simulink model "NeuromuscularModel_3R60_2D"  (R2019b)
settings: Solver=ode15s  StartTime=0.0  StopTime=30  MaxStep=.01  RelTol=1e-4  AbsTol=1e-6  EnableMultiTasking=on
values from neighbouring files (symbols this model uses):
  dt_visual = 1/50    (= 0.02)    [evaluateCost.m]    (also in optimize.m = 0.0333333333333)
  initialTargetAngle = 70*pi/180    (= 1.2217304764)    [setInit.m]
  LongDelay = 0.020    (= 0.02)    [ControlParams.m]
  LPreStimBFSHst = Gains(51)    [assignGains.m]
  LPreStimGASst = Gains(52)    [assignGains.m]
  LPreStimGLUst = Gains(47)    [assignGains.m]
  LPreStimHAMst = Gains(48)    [assignGains.m]
  LPreStimHFLst = Gains(46)    [assignGains.m]
  LPreStimRFst = Gains(49)    [assignGains.m]
  LPreStimSOLst = Gains(53)    [assignGains.m]
  LPreStimTAst = Gains(54)    [assignGains.m]
  LPreStimVASst = Gains(50)    [assignGains.m]
  MidDelay = 0.010    (= 0.01)    [ControlParams.m]
  RPreStimGLUsw = Gains(95)    [assignGains.m]
  RPreStimHAMsw = Gains(96)    [assignGains.m]
  RPreStimHFLsw = Gains(94)    [assignGains.m]
  RPreStimRFsw = Gains(97)    [assignGains.m]
  ShortDelay = 0.005    [ControlParams.m]
  termination_height = 0.5    [ControlParams.m]
  vy0 = paramIC(10)*.2    [setInit.m]
undefined symbols (not defined in the file or in its folder): g, hatLeftHipToCenterDistWidth, hatLeftHipToCG, initialTargetAngleR, LongLoopDelay, LPreStimHABst, LPreStimHADst, magnitude, obstacle_depth, obstacle_height, obstacle_width, obstacle_x, RPreStimHABsw, RPreStimHADsw, thetaHATref, X, Y, y0, Z
libraries: NeuroMuscularLibrary x100, sm_lib x24, nesl_utility x16, simulink x5
(part 3 of 4)

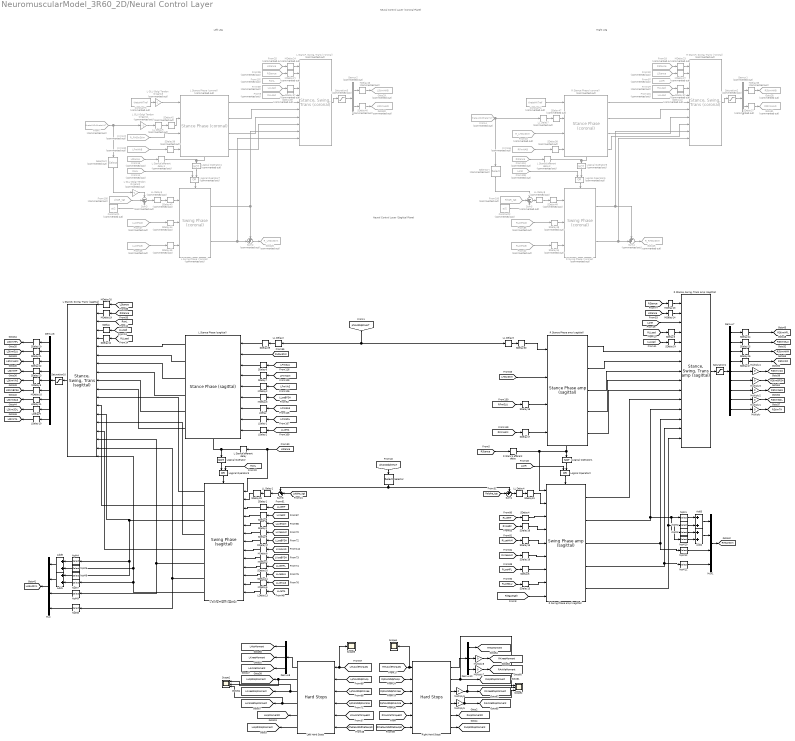
== system NeuromuscularModel_3R60_2D/Neural Control Layer ==
  note: Neural Control Layer
      | (Sagittal Plane)
  note: Neural Control Layer
      | (Coronal Plane)
  note: Right Leg
  note: Left Leg
  Add{1..3,9} (4 alike) : Sum  Inputs=2
  Constant1 : Constant  Commented=on  Value=pi/2
  Constant2 : Constant  Commented=on  Value=pi/2
  Constant3 : Constant  Commented=on  Value=thetaHATref
  Constant4 : Constant  Commented=on  Value=thetaHATref
  Demux1 : Demux  Commented=on  Outputs=2
  Demux10 : Demux  Outputs=3
  Demux2 : Demux  Commented=on  Outputs=2
  Demux6 : Demux  Outputs=9
  Demux7 : Demux  Outputs=9
  Demux8 : Demux  Outputs=3
  From100 : From  Commented=on  GotoTag=RhipR_tgt  TagVisibility=global
      settings: CloseFcn=tagdialog Close
  From101 : From  Commented=on  GotoTag=LLLoad  TagVisibility=global
      settings: CloseFcn=tagdialog Close
  From102 : From  Commented=on  GotoTag=RonL  TagVisibility=global
      settings: CloseFcn=tagdialog Close
  From105 : From  Commented=on  GotoTag=LhipR_tgt  TagVisibility=global
      settings: CloseFcn=tagdialog Close
  From108 : From  Commented=on  GotoTag=LonR  TagVisibility=global
      settings: CloseFcn=tagdialog Close
  From11 : From  Commented=on  GotoTag=RonL  TagVisibility=global
      settings: CloseFcn=tagdialog Close
  From110 : From  Commented=on  GotoTag=RStance  TagVisibility=global
      settings: CloseFcn=tagdialog Close
  From15 : From  Commented=on  GotoTag=LStance  TagVisibility=global
      settings: CloseFcn=tagdialog Close
  From16 : From  Commented=on  GotoTag=R_LHSwStim  TagVisibility=global
      settings: CloseFcn=tagdialog Close
  From18 : From  Commented=on  GotoTag=RStance  TagVisibility=global
      settings: CloseFcn=tagdialog Close
  From22 : From  Commented=on  GotoTag=RLceHAB  TagVisibility=global
      settings: CloseFcn=tagdialog Close
  From23 : From  Commented=on  GotoTag=R_RHSwStim  TagVisibility=global
      settings: CloseFcn=tagdialog Close
  From25 : From  Commented=on  GotoTag=LStance  TagVisibility=global
      settings: CloseFcn=tagdialog Close
  From26 : From  Commented=on  GotoTag=LLceHAB  TagVisibility=global
      settings: CloseFcn=tagdialog Close
  From27 : From  Commented=on  GotoTag=LLceHAD  TagVisibility=global
      settings: CloseFcn=tagdialog Close
  From29 : From  Commented=on  GotoTag=RLLoad  TagVisibility=global
      settings: CloseFcn=tagdialog Close
  From32 : From  Commented=on  GotoTag=LStance  TagVisibility=global
      settings: CloseFcn=tagdialog Close
  From4 : From  Commented=on  GotoTag=thetaANDdthetaHAT  TagVisibility=global
  From7 : From  Commented=on  GotoTag=thetaANDdthetaHAT  TagVisibility=global
  From85 : From  Commented=on  GotoTag=RLceHAD  TagVisibility=global
      settings: CloseFcn=tagdialog Close
  From88 : From  Commented=on  GotoTag=LLLoad  TagVisibility=global
      settings: CloseFcn=tagdialog Close
  From9 : From  Commented=on  GotoTag=RLLoad  TagVisibility=global
      settings: CloseFcn=tagdialog Close
  From94 : From  Commented=on  GotoTag=RFmHAB  TagVisibility=global
      settings: CloseFcn=tagdialog Close
  From95 : From  Commented=on  GotoTag=RStance  TagVisibility=global
      settings: CloseFcn=tagdialog Close
  From97 : From  Commented=on  GotoTag=LonR  TagVisibility=global
      settings: CloseFcn=tagdialog Close
  From99 : From  Commented=on  GotoTag=LFmHAB  TagVisibility=global
      settings: CloseFcn=tagdialog Close
  Goto25 : Goto  Commented=on  GotoTag=R_RHSwStim  TagVisibility=global
  Goto26 : Goto  Commented=on  GotoTag=R_LHSwStim  TagVisibility=global
  Goto28 : Goto  Commented=on  GotoTag=RStimHAB  TagVisibility=global
  Goto29 : Goto  Commented=on  GotoTag=LStimHAB  TagVisibility=global
  Goto30 : Goto  Commented=on  GotoTag=LStimHAD  TagVisibility=global
  Goto31 : Goto  Commented=on  GotoTag=RStimHAD  TagVisibility=global
  L GLU Golgi Tendon Organs1 : Gain  Commented=on  Gain=-1
  L GLU Golgi Tendon Organs2 : Gain  Commented=on  Gain=-1
  L GLU Golgi Tendon Organs3 : Gain  Commented=on  Gain=-1
  L Stance afferent delay : TransportDelay  DelayTime=MidDelay
  L Stance afferent delay1 : TransportDelay  Commented=on  DelayTime=MidDelay
  L Stance afferent delay2 : TransportDelay  Commented=on  DelayTime=MidDelay
  L Stance Phase (coronal) : NeuroMuscularLibrary/Stance Phase (coronal)  Commented=on  PreStimHABst=LPreStimHABst  PreStimHADst=LPreStimHADst  GainFHABst=LGainFHABst  GainPhiHATHABst=LGainPhiHATHABst  GainDphiHATHABst=LGainDphiHATHABst  GainPhiHATHADst=LGainPhiHATHADst  GainDphiHATHADst=LGainDphiHATHADst  GainSHABcHABst=LGainSHABcHABst  GainSHADcHADst=LGainSHADcHADst
  L Stance Phase (sagittal) : NeuroMuscularLibrary/Stance Phase (sagittal)  PreStimHFLst=LPreStimHFLst  PreStimGLUst=LPreStimGLUst  PreStimHAMst=LPreStimHAMst  PreStimRFst=LPreStimRFst  PreStimVASst=LPreStimVASst  PreStimBFSHst=LPreStimBFSHst  PreStimGASst=LPreStimGASst  PreStimSOLst=LPreStimSOLst  PreStimTAst=LPreStimTAst  GainFGLUst=LGainFGLUst  GainFVASst=LGainFVASst  GainFSOLst=LGainFSOLst  GainFHAMst=LGainFHAMst  LceOffsetBFSHVASst=LLceOffsetBFSHVASst  GainLBFSHVASst=LGainLBFSHVASst  LceOffsetBFSHst=LLceOffsetBFSHst  GainLBFSHst=LGainLBFSHst  GainFGASst=LGainFGASst  phiHATref=phiHATref  GainPhiHATHFLst=LGainPhiHATHFLst  GainDphiHATHFLst=LGainDphiHATHFLst  GainPhiHATGLUst=LGainPhiHATGLUst  GainDphiHATGLUst=LGainDphiHATGLUst  GainSGLUHAMst=LGainSGLUHAMst  GainSGLUcHFLst=LGainSGLUcHFLst  GainSHAMcHFLst=LGainSHAMcHFLst  GainSHFLcGLUst=LGainSHFLcGLUst  GainSRFcGLUst=LGainSRFcGLUst  LceOffsetTAst=LLceOffsetTAst  GainLTAst=LGainLTAst  GainFSOLTAst=LGainFSOLTAst
  "L Stance, Swing, Trans (coronal)" : NeuroMuscularLibrary/Stance, Swing, Trans (coronal)  Commented=on  transSupst_C=LtransSupst_C  transsw_C=Ltranssw_C
  "L Stance, Swing, Trans (sagittal)" : NeuroMuscularLibrary/Stance, Swing, Trans (sagittal)  transSupst=LtransSupst  transsw=Ltranssw
  L Swing Phase (coronal) : NeuroMuscularLibrary/Swing Phase (coronal)  Commented=on  PreStimHABsw=LPreStimHABsw  PreStimHADsw=LPreStimHADsw  GainLHABsw=LGainLHABsw  GainLHADsw=LGainLHADsw
  L Swing Phase (sagittal) : NeuroMuscularLibrary/Swing Phase (sagittal)  PreStimHFLsw=LPreStimHFLsw  PreStimGLUsw=LPreStimGLUsw  PreStimHAMsw=LPreStimHAMsw  PreStimRFsw=LPreStimRFsw  PreStimVASsw=LPreStimVASsw  PreStimBFSHsw=LPreStimBFSHsw  PreStimGASsw=LPreStimGASsw  PreStimSOLsw=LPreStimSOLsw  PreStimTAsw=LPreStimTAsw  GainLTAsw=LGainLTAsw  LceOffsetTAsw=LLceOffsetTAsw  GainLRFHFLsw=LGainLRFHFLsw  GainVRFHFLsw=LGainVRFHFLsw  GainLHAMGLUsw=LGainLHAMGLUsw  GainVHAMGLUsw=LGainVHAMGLUsw  GainVRFBFSHsw=LGainVRFBFSHsw  GainVVASRFsw=LGainVVASRFsw  GainVBFSHsw=LGainVBFSHsw  GainLHAMsw=LGainLHAMsw  GainSHAMBFSHsw=LGainSHAMBFSHsw  GainSHAMGASsw=LGainSHAMGASsw  SHAMthresholdsw=LSHAMthresholdsw  GainLHFLsw=LGainLHFLsw  GainLGLUsw=LGainLGLUsw  LceOffsetVASsw=LLceOffsetVASsw  GainLVASsw=LGainLVASsw  legLengthClr=LlegLengthClr  deltaLegAngleThr=LdeltaLegAngleThr
  LDelay : TransportDelay  DelayTime=LongDelay
  LDelay1 : TransportDelay  DelayTime=LongDelay
  LDelay10 : TransportDelay  DelayTime=LongDelay  InitialOutput=LPreStimTAst
  LDelay11 : TransportDelay  DelayTime=LongDelay  InitialOutput=LPreStimGASst
  LDelay13 : TransportDelay  DelayTime=LongDelay  InitialOutput=1
  LDelay2 : TransportDelay  DelayTime=LongDelay  InitialOutput=1
  LDelay9 : TransportDelay  DelayTime=LongDelay  InitialOutput=LPreStimSOLst
  LL Delay1 : TransportDelay  DelayTime=LongLoopDelay/2  InitialOutput=initialTargetAngle
  LL Delay2 : TransportDelay  DelayTime=LongLoopDelay/2
  LL Delay3 : TransportDelay  DelayTime=LongLoopDelay/2
  LL Delay4 : TransportDelay  DelayTime=LongLoopDelay/2  InitialOutput=initialTargetAngle
  LL Delay5 : TransportDelay  Commented=on  DelayTime=LongLoopDelay/2  InitialOutput=initialTargetAngleR
  LL Delay6 : TransportDelay  Commented=on  DelayTime=LongLoopDelay/2
  LL Delay7 : TransportDelay  Commented=on  DelayTime=LongLoopDelay/2
  LL Delay8 : TransportDelay  Commented=on  DelayTime=LongLoopDelay/2  InitialOutput=initialTargetAngleR
  Left Hard Stops : NeuroMuscularLibrary/Hard Stops  SystemSampleTime=-1  Latency=0  AutoFrameSizeCalculation=off
  Logical Operator : Logic  Operator=NOT  AllPortsSameDT=off  OutDataTypeStr=boolean
  Logical Operator1 : Logic  Operator=NOT  AllPortsSameDT=off  OutDataTypeStr=boolean
  Logical Operator2 : Logic  Operator=OR  AllPortsSameDT=off  OutDataTypeStr=boolean
  Logical Operator3 : Logic  Operator=OR  AllPortsSameDT=off  OutDataTypeStr=boolean
  Logical Operator4 : Logic  Commented=on  Operator=NOT  AllPortsSameDT=off  OutDataTypeStr=boolean
  Logical Operator5 : Logic  Commented=on  Operator=NOT  AllPortsSameDT=off  OutDataTypeStr=boolean
  Logical Operator6 : Logic  Commented=on  Operator=OR  AllPortsSameDT=off  OutDataTypeStr=boolean
  Logical Operator7 : Logic  Commented=on  Operator=OR  AllPortsSameDT=off  OutDataTypeStr=boolean
  MDelay10 : TransportDelay  DelayTime=MidDelay  InitialOutput=LPreStimBFSHst
  MDelay{2,4,8,13..14,19..20} (7 alike) : TransportDelay  DelayTime=MidDelay
  MDelay17 : TransportDelay  DelayTime=MidDelay  InitialOutput=1
  MDelay{21..24} (4 alike) : TransportDelay  Commented=on  DelayTime=MidDelay
  MDelay3 : TransportDelay  DelayTime=MidDelay  InitialOutput=1
  MDelay5 : TransportDelay  DelayTime=MidDelay  InitialOutput=1
  MDelay9 : TransportDelay  DelayTime=MidDelay  InitialOutput=LPreStimVASst
  Multiply{,1..8} (9 alike) : Gain  Gain=0
  Mux : Mux
  Mux1 : Mux
  R Stance afferent delay : TransportDelay  DelayTime=MidDelay
  R Stance Phase (coronal) : NeuroMuscularLibrary/Stance Phase (coronal)  Commented=on  PreStimHABst=RPreStimHABst  PreStimHADst=RPreStimHADst  GainFHABst=RGainFHABst  GainPhiHATHABst=RGainPhiHATHABst  GainDphiHATHABst=RGainDphiHATHABst  GainPhiHATHADst=RGainPhiHATHADst  GainDphiHATHADst=RGainDphiHATHADst  GainSHABcHABst=RGainSHABcHABst  GainSHADcHADst=RGainSHADcHADst
  R Stance Phase amp (sagittal) : NeuroMuscularLibrary/Stance Phase amp (sagittal)  PreStimHFLst=RPreStimHFLst  PreStimGLUst=RPreStimGLUst  PreStimHAMst=RPreStimHAMst  PreStimRFst=RPreStimRFst  GainFGLUst=RGainFGLUst  GainFHAMst=RGainFHAMst  phiHATref=phiHATref  GainPhiHATHFLst=RGainPhiHATHFLst  GainDphiHATHFLst=RGainDphiHATHFLst  GainPhiHATGLUst=RGainPhiHATGLUst  GainDphiHATGLUst=RGainDphiHATGLUst  GainSGLUHAMst=RGainSGLUHAMst  GainSGLUcHFLst=RGainSGLUcHFLst  GainSHAMcHFLst=RGainSHAMcHFLst  GainSHFLcGLUst=RGainSHFLcGLUst  GainSRFcGLUst=RGainSRFcGLUst
  "R Stance, Swing, Trans (coronal)" : NeuroMuscularLibrary/Stance, Swing, Trans (coronal)  Commented=on  transSupst_C=RtransSupst_C  transsw_C=Rtranssw_C
  "R Stance, Swing, Trans amp (sagittal)" : NeuroMuscularLibrary/Stance, Swing, Trans amp (sagittal)  transSupst=RtransSupst  transsw=Rtranssw
  R Swing Phase (coronal) : NeuroMuscularLibrary/Swing Phase (coronal)  Commented=on  PreStimHABsw=RPreStimHABsw  PreStimHADsw=RPreStimHADsw  GainLHABsw=RGainLHABsw  GainLHADsw=RGainLHADsw
  R Swing Phase amp (sagittal) : NeuroMuscularLibrary/Swing Phase amp (sagittal)  PreStimHFLsw=RPreStimHFLsw  PreStimGLUsw=RPreStimGLUsw  PreStimHAMsw=RPreStimHAMsw  PreStimRFsw=RPreStimRFsw  GainLRFHFLsw=RGainLRFHFLsw  GainVRFHFLsw=RGainVRFHFLsw  GainLHAMGLUsw=RGainLHAMGLUsw  GainVHAMGLUsw=RGainVHAMGLUsw  GainLHAMsw=RGainLHAMsw  GainLHFLsw=RGainLHFLsw  GainLGLUsw=RGainLGLUsw  legLengthClr=RlegLengthClr  deltaLegAngleThr=RdeltaLegAngleThr
  Right Hard Stops : NeuroMuscularLibrary/Hard Stops  SystemSampleTime=-1  Latency=0  AutoFrameSizeCalculation=off
  SDelay{,3,6..9,12,14,16..19,29..30} (14 alike) : TransportDelay  DelayTime=ShortDelay
  SDelay{1..2,4..5,10..11,13,15} (8 alike) : TransportDelay  DelayTime=ShortDelay  InitialOutput=1
  SDelay20 : TransportDelay  DelayTime=ShortDelay  InitialOutput=LPreStimHFLst
  SDelay21 : TransportDelay  DelayTime=ShortDelay  InitialOutput=LPreStimGLUst
  SDelay22 : TransportDelay  DelayTime=ShortDelay  InitialOutput=LPreStimHAMst
  SDelay23 : TransportDelay  DelayTime=ShortDelay  InitialOutput=LPreStimRFst
  SDelay24 : TransportDelay  DelayTime=ShortDelay  InitialOutput=RPreStimHFLsw
  SDelay25 : TransportDelay  DelayTime=ShortDelay  InitialOutput=RPreStimGLUsw
  SDelay26 : TransportDelay  DelayTime=ShortDelay  InitialOutput=RPreStimHAMsw
  SDelay27 : TransportDelay  DelayTime=ShortDelay  InitialOutput=RPreStimRFsw
  SDelay28 : TransportDelay  DelayTime=ShortDelay  InitialOutput=initialTargetAngle
  SDelay31 : TransportDelay  DelayTime=ShortDelay  InitialOutput=initialTargetAngle
  SDelay{32..33,36,38..39,41..42,47} (8 alike) : TransportDelay  Commented=on  DelayTime=ShortDelay
  SDelay{34,44..45,49} (4 alike) : TransportDelay  Commented=on  DelayTime=ShortDelay  InitialOutput=1
  SDelay35 : TransportDelay  Commented=on  DelayTime=ShortDelay  InitialOutput=RPreStimHABsw
  SDelay37 : TransportDelay  Commented=on  DelayTime=ShortDelay  InitialOutput=RPreStimHADsw
  SDelay40 : TransportDelay  Commented=on  DelayTime=ShortDelay  InitialOutput=LPreStimHADst
  SDelay43 : TransportDelay  Commented=on  DelayTime=ShortDelay  InitialOutput=initialTargetAngleR
  SDelay46 : TransportDelay  Commented=on  DelayTime=ShortDelay  InitialOutput=LPreStimHABst
  SDelay48 : TransportDelay  Commented=on  DelayTime=ShortDelay  InitialOutput=initialTargetAngleR
  Saturation1 : Saturate  UpperLimit=1  LowerLimit=0.01  ZeroCross=off
  Saturation10 : Saturate  UpperLimit=1  LowerLimit=0.01  ZeroCross=off
  Saturation2 : Saturate  Commented=on  UpperLimit=1  LowerLimit=0.01  ZeroCross=off
  Saturation3 : Saturate  Commented=on  UpperLimit=1  LowerLimit=0.01  ZeroCross=off
  Scope1 : Scope  NumInputPorts=3
  Scope2 : Scope  NumInputPorts=3
  Scope3 : Scope
  Scope4 : Scope
  Selector : Selector  InputPortWidth=2  IndexOptions=Index vector (dialog)  Indices=[1]  OutputSizes=1
  Selector1 : Selector  Commented=on  InputPortWidth=2  IndexOptions=Index vector (dialog)  Indices=[1]  OutputSizes=1
  Selector2 : Selector  Commented=on  InputPortWidth=2  IndexOptions=Index vector (dialog)  Indices=[1]  OutputSizes=1
  Sum1 : Sum  Inputs=-+|
  Sum2 : Sum  Commented=on  Inputs=++|
  Sum3 : Sum  Commented=on  Inputs=--+
  Sum4 : Sum  Commented=on  Inputs=++|
  Sum5 : Sum  Commented=on  Inputs=--+
  Sum6 : Sum  Inputs=-+|
  hipM{1,4,9,12} (4 alike) : Selector  InputPortWidth=2  IndexOptions=Index vector (dialog)  Indices=1  OutputSizes=1
  hipM10 : Selector  InputPortWidth=3  IndexOptions=Index vector (dialog)  Indices=2  OutputSizes=1
  hipM{2,5,8,11} (4 alike) : Selector  InputPortWidth=3  IndexOptions=Index vector (dialog)  Indices=1  OutputSizes=1
  hipM3 : Selector  InputPortWidth=2  IndexOptions=Index vector (dialog)  Indices=2  OutputSizes=1
  hipM6 : Selector  InputPortWidth=2  IndexOptions=Index vector (dialog)  Indices=2  OutputSizes=1
  hipM7 : Selector  InputPortWidth=3  IndexOptions=Index vector (dialog)  Indices=2  OutputSizes=1
  tag scope: LAnkleMoment=global, LAnkleStopMoment=global, LHSwStim=global, LHipMoment=global, LHipMomentR=global, LHipRStopMoment=global, LHipStopMoment=global, LKneeMoment=global, LKneeStopMoment=global, LStimBFSH=global, LStimGAS=global, LStimGLU=global, LStimHAM=global, LStimHFL=global, LStimRF=global, LStimSOL=global, LStimTA=global, LStimVAS=global, RAnkleMoment=global, RAnkleStopMoment=global, RHSwStim=global, RHipMoment=global, RHipMomentR=global, RHipRStopMoment=global, RHipStopMoment=global, RKneeMoment=global, RKneeStopMoment=global, RStimBFSH=global, RStimGAS=global, RStimGLU=global, RStimHAM=global, RStimHFL=global, RStimRF=global, RStimSOL=global, RStimTA=global, RStimVAS=global
  wires:
  LDelay11/1 -> [LStimGAS]
  LDelay10/1 -> [LStimTA]
  L Swing Phase (sagittal)/7 -> "L Stance, Swing, Trans (sagittal)"/18, hipM8/1
  Mux/1 -> [LHSwStim]
  hipM2/1 -> Add3/2
  SDelay11/1 -> L Swing Phase (sagittal)/11
  SDelay24/1 -> [RStimHFL]
  [RLceRF] -> SDelay4/1
  MDelay19/1 -> "L Stance, Swing, Trans (sagittal)"/2
  SDelay10/1 -> L Swing Phase (sagittal)/10
  hipM10/1 -> Add2/2
  R Stance Phase amp (sagittal)/5 -> "R Stance, Swing, Trans amp (sagittal)"/10
  hipM4/1 -> Add9/1
  SDelay2/1 -> L Swing Phase (sagittal)/5
  [RLceGLU] -> SDelay13/1
  L Swing Phase (sagittal)/1 -> "L Stance, Swing, Trans (sagittal)"/12
  LDelay/1 -> L Stance Phase (sagittal)/7
  L Stance Phase (sagittal)/1 -> "L Stance, Swing, Trans (sagittal)"/6
  SDelay9/1 -> L Swing Phase (sagittal)/6
  L Swing Phase (sagittal)/3 -> "L Stance, Swing, Trans (sagittal)"/14, hipM6/1, hipM4/1
  R Swing Phase amp (sagittal)/4 -> "R Stance, Swing, Trans amp (sagittal)"/14, hipM11/1
  Add2/1 -> Mux1/2
  L Swing Phase (sagittal)/5 -> "L Stance, Swing, Trans (sagittal)"/16
  SDelay14/1 -> "R Stance, Swing, Trans amp (sagittal)"/5
  Demux6/2 -> SDelay21/1
  R Stance Phase amp (sagittal)/2 -> "R Stance, Swing, Trans amp (sagittal)"/7
  SDelay12/1 -> "L Stance, Swing, Trans (sagittal)"/5
  MDelay2/1 -> L Stance Phase (sagittal)/5
  Sum1/1 -> LL Delay4/1
  hipM6/1 -> Add1/1
  R Stance Phase amp (sagittal)/3 -> "R Stance, Swing, Trans amp (sagittal)"/8
  LDelay9/1 -> [LStimSOL]
  Demux6/1 -> SDelay20/1
  L Stance Phase (sagittal)/6 -> "L Stance, Swing, Trans (sagittal)"/11
  SDelay4/1 -> R Swing Phase amp (sagittal)/3
  hipM11/1 -> Mux1/4
  MDelay8/1 -> L Swing Phase (sagittal)/8
  Add3/1 -> Mux1/1
  R Swing Phase amp (sagittal)/3 -> "R Stance, Swing, Trans amp (sagittal)"/13, hipM12/1
  "R Stance, Swing, Trans amp (sagittal)"/1 -> Saturation1/1
  Add1/1 -> Mux/2
  hipM9/1 -> Mux/3
  L Stance Phase (sagittal)/3 -> "L Stance, Swing, Trans (sagittal)"/8
  Demux7/8 -> Multiply1/1
  Logical Operator2/1 -> R Swing Phase amp (sagittal)/Enable
  hipM5/1 -> Add9/2
  MDelay20/1 -> "L Stance, Swing, Trans (sagittal)"/1
  L Swing Phase (sagittal)/2 -> "L Stance, Swing, Trans (sagittal)"/13
  hipM8/1 -> Mux/4
  L Swing Phase (sagittal)/4 -> "L Stance, Swing, Trans (sagittal)"/15
  L Swing Phase (sagittal)/8 -> "L Stance, Swing, Trans (sagittal)"/19, hipM5/1, hipM7/1
  [LStance] -> MDelay20/1
  R Stance Phase amp (sagittal)/4 -> "R Stance, Swing, Trans amp (sagittal)"/9
  LL Delay3/1 -> SDelay30/1
  SDelay30/1 -> R Stance Phase amp (sagittal)/1
  SDelay22/1 -> [LStimHAM]
  SDelay29/1 -> L Stance Phase (sagittal)/1
  SDelay28/1 -> L Swing Phase (sagittal)/2
  hipM1/1 -> Add3/1
  R Swing Phase amp (sagittal)/5 -> "R Stance, Swing, Trans amp (sagittal)"/15, hipM2/1, hipM10/1
  Sum6/1 -> LL Delay1/1
  Demux7/1 -> SDelay24/1
  [LLceGLU] -> SDelay11/1
  [RLceHFL] -> SDelay5/1
  LL Delay4/1 -> SDelay31/1
  L Stance Phase (sagittal)/2 -> "L Stance, Swing, Trans (sagittal)"/7
  R Stance Phase amp (sagittal)/1 -> "R Stance, Swing, Trans amp (sagittal)"/6
  [LLceVAS] -> MDelay5/1
  [LHSwStim] -> R Stance Phase amp (sagittal)/2
  SDelay/1 -> "L Stance, Swing, Trans (sagittal)"/4
  SDelay27/1 -> [RStimRF]
  Demux7/6 -> Multiply3/1
  MDelay10/1 -> [LStimBFSH]
  Add9/1 -> Mux/1
  [LLceHFL] -> SDelay10/1
  SDelay26/1 -> [RStimHAM]
  SDelay21/1 -> [LStimGLU]
  [LLLoad] -> SDelay14/1
  Saturation1/1 -> Demux7/1
  SDelay5/1 -> R Swing Phase amp (sagittal)/7
  [LFmSOL] -> LDelay1/1
  hipM12/1 -> Mux1/3
  [LonR] -> "R Stance, Swing, Trans amp (sagittal)"/3
  [LLLoad] -> SDelay/1
  SDelay25/1 -> [RStimGLU]
  Demux7/3 -> SDelay26/1
  L Stance Phase (sagittal)/4 -> "L Stance, Swing, Trans (sagittal)"/9
  Demux7/4 -> SDelay27/1
  hipM3/1 -> Add2/1
  R Swing Phase amp (sagittal)/1 -> "R Stance, Swing, Trans amp (sagittal)"/11
  L Stance Phase (sagittal)/5 -> "L Stance, Swing, Trans (sagittal)"/10
  LL Delay1/1 -> SDelay28/1
  MDelay9/1 -> [LStimVAS]
  SDelay3/1 -> "R Stance, Swing, Trans amp (sagittal)"/4
  SDelay31/1 -> R Swing Phase amp (sagittal)/2
  SDelay19/1 -> R Swing Phase amp (sagittal)/6
  [RVceHAM] -> SDelay19/1
  SDelay18/1 -> R Swing Phase amp (sagittal)/4
  SDelay15/1 -> R Swing Phase amp (sagittal)/5
  [RLceHAM] -> SDelay15/1
  Demux7/7 -> Multiply2/1
  [LLceBFSH] -> MDelay3/1
  [RLLoad] -> SDelay3/1
  SDelay17/1 -> R Stance Phase amp (sagittal)/4
  Demux6/7 -> LDelay11/1
  [RStance] -> MDelay19/1
  Saturation10/1 -> Demux6/1
  MDelay4/1 -> L Swing Phase (sagittal)/9
  L Swing Phase (sagittal)/6 -> "L Stance, Swing, Trans (sagittal)"/17, hipM9/1
  Demux6/6 -> MDelay10/1
  Demux6/3 -> SDelay22/1
  Demux7/9 -> Multiply/1
  [LVceBFSH] -> MDelay4/1
  SDelay8/1 -> L Swing Phase (sagittal)/4
  Demux6/9 -> LDelay10/1
  [RVceRF] -> SDelay18/1
  Demux6/8 -> LDelay9/1
  Demux6/5 -> MDelay9/1
  MDelay5/1 -> L Swing Phase (sagittal)/12
  SDelay16/1 -> R Stance Phase amp (sagittal)/3
  SDelay23/1 -> [LStimRF]
  [RLLoad] -> SDelay12/1
  R Swing Phase amp (sagittal)/2 -> "R Stance, Swing, Trans amp (sagittal)"/12, hipM3/1, hipM1/1
  [LVceRF] -> SDelay8/1
  SDelay13/1 -> R Swing Phase amp (sagittal)/8
  Mux1/1 -> [RHSwStim]
  L Stance afferent delay/1 -> L Stance Phase (sagittal)/Enable, Logical Operator/1
  Logical Operator3/1 -> L Swing Phase (sagittal)/Enable
  SDelay20/1 -> [LStimHFL]
  [LLceRF] -> SDelay1/1
  [LVceHAM] -> SDelay9/1
  LDelay2/1 -> L Stance Phase (sagittal)/9
  [LLceTA] -> LDelay2/1
  Demux7/2 -> SDelay25/1
  SDelay1/1 -> L Swing Phase (sagittal)/3
  [RFmHAM] -> SDelay17/1
  Logical Operator/1 -> Logical Operator3/2
  [LLceHAM] -> SDelay2/1
  Demux6/4 -> SDelay23/1
  LDelay1/1 -> L Stance Phase (sagittal)/8
  [LFmGAS] -> LDelay/1
  [RFmGLU] -> SDelay16/1
  MDelay3/1 -> L Stance Phase (sagittal)/6
  SDelay6/1 -> L Stance Phase (sagittal)/3
  [LVceVAS] -> MDelay8/1
  [LFmVAS] -> MDelay2/1
  LL Delay2/1 -> SDelay29/1
  [LFmGLU] -> SDelay6/1
  SDelay7/1 -> L Stance Phase (sagittal)/4
  Demux7/5 -> Multiply4/1
  [LFmHAM] -> SDelay7/1
  [RHSwStim] -> L Stance Phase (sagittal)/2
  hipM7/1 -> Add1/2
  Logical Operator1/1 -> Logical Operator2/2
  [LLceTA] -> LDelay13/1
  MDelay17/1 -> L Swing Phase (sagittal)/7
  [LLceBFSH] -> MDelay17/1
  LDelay13/1 -> L Swing Phase (sagittal)/13
  R Stance afferent delay/1 -> R Swing Phase amp (sagittal)/1, R Stance Phase amp (sagittal)/Enable, Logical Operator1/1
  [RonL] -> "L Stance, Swing, Trans (sagittal)"/3
  [LonR] -> Logical Operator2/1
  [RonL] -> Logical Operator3/1
  [RStance] -> MDelay13/1
  MDelay13/1 -> "R Stance, Swing, Trans amp (sagittal)"/1
  [LStance] -> MDelay14/1
  MDelay14/1 -> "R Stance, Swing, Trans amp (sagittal)"/2
  [Ralpha_tgt] -> Sum1/2
  Selector/1 -> Sum6/1, Sum1/1
  [Lalpha_tgt] -> Sum6/2
  [phiANDdphiHAT] -> LL Delay2/1, LL Delay3/1
  From94/1 -> SDelay38/1
  SDelay35/1 -> Goto28/1
  From99/1 -> SDelay39/1
  SDelay37/1 -> Goto31/1
  From27/1 -> SDelay44/1
  SDelay39/1 -> L Stance Phase (coronal)/4
  L Stance Phase (coronal)/2 -> "L Stance, Swing, Trans (coronal)"/7
  MDelay21/1 -> "L Stance, Swing, Trans (coronal)"/2
  L Swing Phase (coronal)/2 -> "L Stance, Swing, Trans (coronal)"/11, Sum2/2
  From105/1 -> Sum3/2
  L GLU Golgi Tendon Organs2/1 -> Sum3/1
  Logical Operator5/1 -> Logical Operator6/2
  From85/1 -> SDelay49/1
  Selector2/1 -> L GLU Golgi Tendon Organs2/1
  Logical Operator4/1 -> Logical Operator7/2
  From26/1 -> SDelay45/1
  Constant4/1 -> R Stance Phase (coronal)/1
  From11/1 -> Logical Operator7/1
  Logical Operator6/1 -> R Swing Phase (coronal)/Enable
  L Swing Phase (coronal)/1 -> "L Stance, Swing, Trans (coronal)"/10, Sum2/1
  L Stance Phase (coronal)/1 -> "L Stance, Swing, Trans (coronal)"/6
  SDelay32/1 -> "L Stance, Swing, Trans (coronal)"/4
  L GLU Golgi Tendon Organs1/1 -> LL Delay6/1
  Sum3/1 -> LL Delay5/1
  "L Stance, Swing, Trans (coronal)"/1 -> Saturation3/1
  SDelay43/1 -> L Swing Phase (coronal)/1
  SDelay40/1 -> Goto30/1
  MDelay24/1 -> "L Stance, Swing, Trans (coronal)"/1
  Selector1/1 -> Sum5/1
  L Stance afferent delay1/1 -> L Stance Phase (coronal)/Enable, Logical Operator4/1
  SDelay46/1 -> Goto29/1
  LL Delay5/1 -> SDelay43/1
  SDelay45/1 -> L Swing Phase (coronal)/3
  SDelay44/1 -> L Swing Phase (coronal)/2
  From18/1 -> MDelay23/1
  MDelay23/1 -> "R Stance, Swing, Trans (coronal)"/1
  SDelay49/1 -> R Swing Phase (coronal)/2
  From16/1 -> R Stance Phase (coronal)/3
  LL Delay8/1 -> SDelay48/1
  Logical Operator7/1 -> L Swing Phase (coronal)/Enable
  Sum2/1 -> Goto26/1
  From15/1 -> L Stance afferent delay1/1
  L Stance Phase (coronal)/4 -> "L Stance, Swing, Trans (coronal)"/9
  Demux1/2 -> SDelay37/1
  SDelay42/1 -> L Stance Phase (coronal)/2
  From102/1 -> "L Stance, Swing, Trans (coronal)"/3
  L Stance afferent delay2/1 -> R Stance Phase (coronal)/Enable, Logical Operator5/1
  L Stance Phase (coronal)/3 -> "L Stance, Swing, Trans (coronal)"/8
  SDelay36/1 -> "L Stance, Swing, Trans (coronal)"/5
  Demux2/1 -> SDelay46/1
  From88/1 -> SDelay32/1
  From95/1 -> MDelay21/1
  From29/1 -> SDelay33/1
  From110/1 -> L Stance afferent delay2/1
  From25/1 -> MDelay24/1
  From101/1 -> SDelay41/1
  From108/1 -> Logical Operator6/1
  From9/1 -> SDelay36/1
  From23/1 -> L Stance Phase (coronal)/3
  L GLU Golgi Tendon Organs3/1 -> L Stance Phase (coronal)/1
  SDelay41/1 -> "R Stance, Swing, Trans (coronal)"/5
  "R Stance, Swing, Trans (coronal)"/1 -> Saturation2/1
  SDelay47/1 -> R Stance Phase (coronal)/2
  Constant2/1 -> Sum5/3
  R Stance Phase (coronal)/2 -> "R Stance, Swing, Trans (coronal)"/7
  SDelay38/1 -> R Stance Phase (coronal)/4
  Saturation2/1 -> Demux1/1
  From32/1 -> MDelay22/1
  SDelay34/1 -> R Swing Phase (coronal)/3
  Sum5/1 -> LL Delay8/1
  MDelay22/1 -> "R Stance, Swing, Trans (coronal)"/2
  Constant1/1 -> Sum3/3
  From97/1 -> "R Stance, Swing, Trans (coronal)"/3
  SDelay48/1 -> R Swing Phase (coronal)/1
  From22/1 -> SDelay34/1
  R Stance Phase (coronal)/1 -> "R Stance, Swing, Trans (coronal)"/6
  Saturation3/1 -> Demux2/1
  R Swing Phase (coronal)/1 -> "R Stance, Swing, Trans (coronal)"/10, Sum4/1
  LL Delay7/1 -> SDelay47/1
  R Stance Phase (coronal)/3 -> "R Stance, Swing, Trans (coronal)"/8
  LL Delay6/1 -> SDelay42/1
  R Stance Phase (coronal)/4 -> "R Stance, Swing, Trans (coronal)"/9
  Demux1/1 -> SDelay35/1
  Demux2/2 -> SDelay40/1
  R Swing Phase (coronal)/2 -> "R Stance, Swing, Trans (coronal)"/11, Sum4/2
  SDelay33/1 -> "R Stance, Swing, Trans (coronal)"/4
  Sum4/1 -> Goto25/1
  From100/1 -> Sum5/2
  Constant3/1 -> L GLU Golgi Tendon Organs3/1
  "L Stance, Swing, Trans (sagittal)"/1 -> Saturation10/1
  [RphiANDdphiHip] -> Right Hard Stops/2
  Demux10/2 -> Multiply8/1
  [RphiANDdphiAnkle] -> Right Hard Stops/4
  [LMuscleTorques] -> Scope3/1, Left Hard Stops/1
  [LphiANDdphiAnkle] -> Left Hard Stops/4
  [LphiANDdphiKnee] -> Left Hard Stops/3
  [RMuscleTorques] -> Scope4/1, Right Hard Stops/1
  [LphiANDdphiHip] -> Left Hard Stops/2
  Right Hard Stops/1 -> Demux10/1
  Left Hard Stops/1 -> Demux8/1
  Right Hard Stops/3 -> Multiply6/1
  Demux10/1 -> [RHipMoment]
  Demux10/3 -> Multiply7/1
  Left Hard Stops/4 -> Scope1/3, [LAnkleStopMoment]
  Right Hard Stops/2 -> Scope2/1, [RHipStopMoment]
  Left Hard Stops/3 -> [LKneeStopMoment], Scope1/2
  Right Hard Stops/4 -> Multiply5/1
  Demux8/2 -> [LKneeMoment]
  Left Hard Stops/2 -> Scope1/1, [LHipStopMoment]
  Demux8/1 -> [LHipMoment]
  Demux8/3 -> [LAnkleMoment]
  [RphiANDdphiKnee] -> Right Hard Stops/3
  [LMuscleTorquesR] -> Left Hard Stops/5
  [RMuscleTorquesR] -> Right Hard Stops/5
  Left Hard Stops/5 -> [LHipMomentR]
  Right Hard Stops/5 -> [RHipMomentR]
  [LthetaANDdthetaHipR] -> Left Hard Stops/6
  [RthetaANDdthetaHipR] -> Right Hard Stops/6
  Left Hard Stops/6 -> [LHipRStopMoment]
  Right Hard Stops/6 -> [RHipRStopMoment]
  [phiANDdphiHAT] -> Selector/1
  From4/1 -> LL Delay7/1, Selector1/1
  From7/1 -> L GLU Golgi Tendon Organs1/1, Selector2/1
  [LStance] -> L Swing Phase (sagittal)/1, L Stance afferent delay/1
  [RStance] -> R Stance afferent delay/1
  Multiply/1 -> [RStimTA]
  Multiply1/1 -> [RStimSOL]
  Multiply2/1 -> [RStimGAS]
  Multiply3/1 -> [RStimBFSH]
  Multiply4/1 -> [RStimVAS]
  [RlegLength] -> R Swing Phase amp (sagittal)/9
  Multiply5/1 -> Scope2/3, [RAnkleStopMoment]
  Multiply6/1 -> Scope2/2, [RKneeStopMoment]
  Multiply7/1 -> [RAnkleMoment]
  Multiply8/1 -> [RKneeMoment]

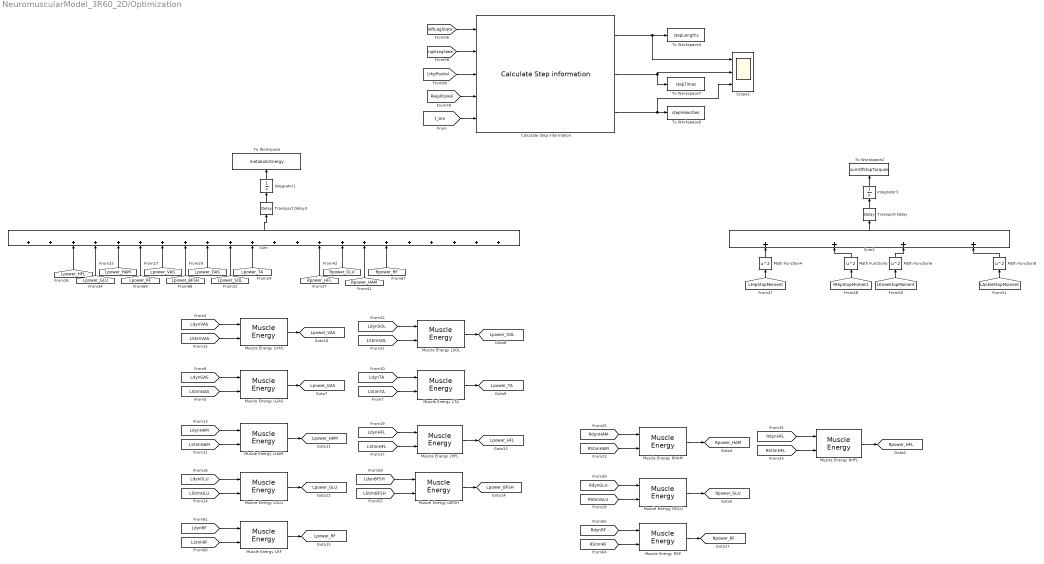
== system NeuromuscularModel_3R60_2D/Optimization ==
  Calculate Step information : NeuroMuscularLibrary/Calculate Step information  SystemSampleTime=-1  Latency=0  AutoFrameSizeCalculation=off
  Integrator1 : Integrator
  Integrator3 : Integrator
  Math Function{4..6,8} (4 alike) : Math  Operator=square  SaturateOnIntegerOverflow=on
  Muscle Energy LBFSH : NeuroMuscularLibrary/Muscle Energy  lopt=loptBFSH  FT=FT_BFSH  Fmax=FmaxBFSH  vmax=vmaxBFSH
  Muscle Energy LGAS : NeuroMuscularLibrary/Muscle Energy  lopt=loptGAS  FT=FT_GAS  Fmax=FmaxGAS  vmax=vmaxGAS
  Muscle Energy LGLU : NeuroMuscularLibrary/Muscle Energy  lopt=loptGLU  FT=FT_GLU  Fmax=FmaxGLU  vmax=vmaxGLU
  Muscle Energy LHAM : NeuroMuscularLibrary/Muscle Energy  lopt=loptHAM  FT=FT_HAM  Fmax=FmaxHAM  vmax=vmaxHAM
  Muscle Energy LHFL : NeuroMuscularLibrary/Muscle Energy  lopt=loptHFL  FT=FT_HFL  Fmax=FmaxHFL  vmax=vmaxHFL
  Muscle Energy LRF : NeuroMuscularLibrary/Muscle Energy  lopt=loptRF  FT=FT_RF  Fmax=FmaxRF  vmax=vmaxRF
  Muscle Energy LSOL : NeuroMuscularLibrary/Muscle Energy  lopt=loptSOL  FT=FT_SOL  Fmax=FmaxSOL  vmax=vmaxSOL
  Muscle Energy LTA : NeuroMuscularLibrary/Muscle Energy  lopt=loptTA  FT=FT_TA  Fmax=FmaxTA  vmax=vmaxTA
  Muscle Energy LVAS : NeuroMuscularLibrary/Muscle Energy  lopt=loptVAS  FT=FT_VAS  Fmax=FmaxVAS  vmax=vmaxVAS
  Muscle Energy RGLU : NeuroMuscularLibrary/Muscle Energy  lopt=loptGLUamp  FT=FT_GLUamp  Fmax=FmaxGLUamp  vmax=vmaxGLUamp
  Muscle Energy RHAM : NeuroMuscularLibrary/Muscle Energy  lopt=loptHAMamp  FT=FT_HAMamp  Fmax=FmaxHAMamp  vmax=vmaxHAMamp
  Muscle Energy RHFL : NeuroMuscularLibrary/Muscle Energy  lopt=loptHFLamp  FT=FT_HFLamp  Fmax=FmaxHFLamp  vmax=vmaxHFLamp
  Muscle Energy RRF : NeuroMuscularLibrary/Muscle Energy  lopt=loptRFamp  FT=FT_RFamp  Fmax=FmaxRFamp  vmax=vmaxRFamp
  Scope1 : Scope  NumInputPorts=3
  Sum : Sum  Inputs=++++++++++++++++++++++
  Sum2 : Sum  Inputs=++++
  To Workspace : ToWorkspace  VariableName=metabolicEnergy  SampleTime=-1
      settings: MaxDataPoints=1
  To Workspace2 : ToWorkspace  VariableName=sumOfStopTorques  SampleTime=-1
      settings: MaxDataPoints=1
  To Workspace4 : ToWorkspace  VariableName=stepLengths  SampleTime=-1
  To Workspace6 : ToWorkspace  VariableName=stepVelocities  SampleTime=-1
  To Workspace7 : ToWorkspace  VariableName=stepTimes  SampleTime=-1
  Transport Delay : TransportDelay  DelayTime=3  BufferSize=24576
  Transport Delay3 : TransportDelay  DelayTime=3  BufferSize=24576
  tag scope: Lpower_BFSH=global, Lpower_GAS=global, Lpower_GLU=global, Lpower_HAM=global, Lpower_HFL=global, Lpower_RF=global, Lpower_SOL=global, Lpower_TA=global, Lpower_VAS=global, Rpower_GLU=global, Rpower_HAM=global, Rpower_HFL=global, Rpower_RF=global
  wires:
  [RdynHAM] -> Muscle Energy RHAM/1
  [RStimHAM] -> Muscle Energy RHAM/2
  [RdynGLU] -> Muscle Energy RGLU/1
  [RStimGLU] -> Muscle Energy RGLU/2
  [RdynHFL] -> Muscle Energy RHFL/1
  [RStimHFL] -> Muscle Energy RHFL/2
  Muscle Energy RHAM/1 -> [Rpower_HAM]
  Muscle Energy RGLU/1 -> [Rpower_GLU]
  Muscle Energy RHFL/1 -> [Rpower_HFL]
  [Lpower_VAS] -> Sum/7
  [Lpower_RF] -> Sum/6
  [Lpower_HAM] -> Sum/5
  [Lpower_GLU] -> Sum/4
  [Lpower_HFL] -> Sum/3
  [LdynSOL] -> Muscle Energy LSOL/1
  [LStimSOL] -> Muscle Energy LSOL/2
  [LStimVAS] -> Muscle Energy LVAS/2
  [LStimGAS] -> Muscle Energy LGAS/2
  Muscle Energy LVAS/1 -> [Lpower_VAS]
  Muscle Energy LGAS/1 -> [Lpower_GAS]
  Muscle Energy LSOL/1 -> [Lpower_SOL]
  Muscle Energy LTA/1 -> [Lpower_TA]
  [LdynTA] -> Muscle Energy LTA/1
  [LStimTA] -> Muscle Energy LTA/2
  [LdynHAM] -> Muscle Energy LHAM/1
  [LStimHAM] -> Muscle Energy LHAM/2
  [LdynGLU] -> Muscle Energy LGLU/1
  [LStimGLU] -> Muscle Energy LGLU/2
  [LdynHFL] -> Muscle Energy LHFL/1
  [LStimHFL] -> Muscle Energy LHFL/2
  Muscle Energy LHAM/1 -> [Lpower_HAM]
  Muscle Energy LGLU/1 -> [Lpower_GLU]
  Muscle Energy LHFL/1 -> [Lpower_HFL]
  [LdynGAS] -> Muscle Energy LGAS/1
  [LdynVAS] -> Muscle Energy LVAS/1
  [Lpower_SOL] -> Sum/10
  [Rpower_HAM] -> Sum/16
  [Rpower_GLU] -> Sum/15
  [Rpower_HFL] -> Sum/14
  [Lpower_TA] -> Sum/11
  Integrator1/1 -> To Workspace/1
  Sum/1 -> Transport Delay3/1
  Integrator3/1 -> To Workspace2/1
  Math Function4/1 -> Sum2/1
  [LHipStopMoment] -> Math Function4/1
  Math Function5/1 -> Sum2/2
  [RHipStopMoment] -> Math Function5/1
  Math Function6/1 -> Sum2/3
  [LKneeStopMoment] -> Math Function6/1
  [LAnkleStopMoment] -> Math Function8/1
  Math Function8/1 -> Sum2/4
  ? -> ?
  Transport Delay/1 -> Integrator3/1
  Sum2/1 -> Transport Delay/1
  Transport Delay3/1 -> Integrator1/1
  [rightLegState] -> Calculate Step information/2
  Calculate Step information/1 -> Scope1/1, To Workspace4/1
  Calculate Step information/3 -> To Workspace6/1, Scope1/3
  Calculate Step information/2 -> To Workspace7/1, Scope1/2
  [leftLegState] -> Calculate Step information/1
  [t_sim] -> Calculate Step information/5
  Muscle Energy LBFSH/1 -> [Lpower_BFSH]
  [LStimBFSH] -> Muscle Energy LBFSH/2
  [LdynBFSH] -> Muscle Energy LBFSH/1
  [LdynRF] -> Muscle Energy LRF/1
  [LStimRF] -> Muscle Energy LRF/2
  Muscle Energy LRF/1 -> [Lpower_RF]
  Muscle Energy RRF/1 -> [Rpower_RF]
  [RdynRF] -> Muscle Energy RRF/1
  [RStimRF] -> Muscle Energy RRF/2
  [Lpower_BFSH] -> Sum/8
  [Lpower_GAS] -> Sum/9
  [Rpower_RF] -> Sum/17
  [RHipPosVel] -> Calculate Step information/4
  [LHipPosVel] -> Calculate Step information/3

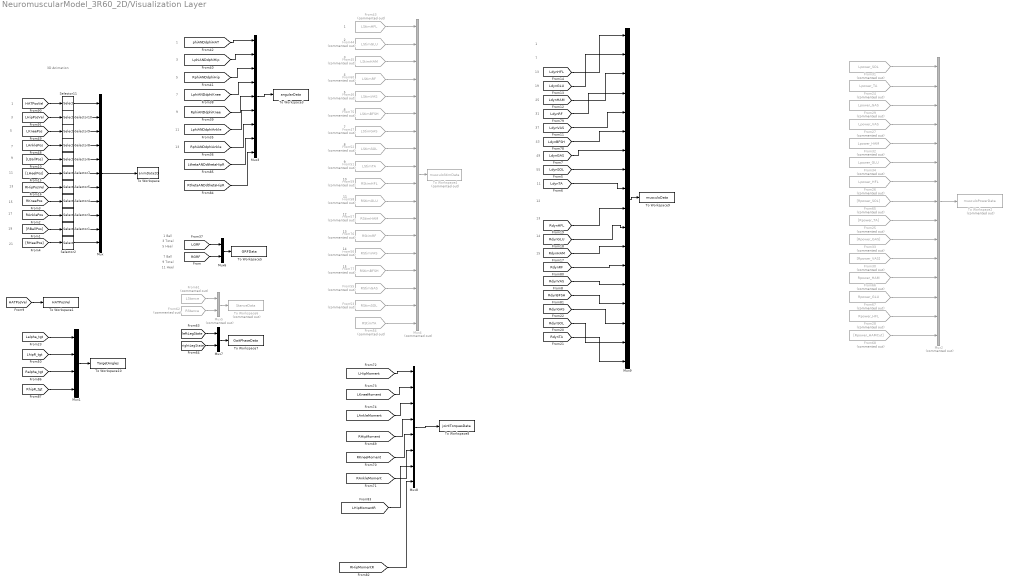
== system NeuromuscularModel_3R60_2D/Visualization Layer ==
  note: 21
  note: 19
  note: 17
  note: 15
  note: 13
  note: 11
  note: 9
  note: 7
  note: 5
  note: 3
  note: 1
  note: 3D Animation
  note: 1
  note: 8
  note: 13
  note: 3
  note: 1
  note: 5
  note: 10
  note: 4
  note: 6
  note: 3
  note: 5
  note: 7
  note: 9
  note: 9
  note: 11
  note: 2
  note: 7
  note: 11
  note: 12
  note: 15
  note: 9 Total
  note: 1 Ball
  note: 5 Heel
  note: 14
  note: 11 Heel
  note: 3 Total
  note: 13
  note: 7 Ball
  note: 7
  note: 12
  note: 13
  note: 55
  note: 14
  note: 19
  note: 1
  note: 43
  note: 49
  note: 37
  note: 25
  note: 11
  note: 13
  note: 15
  note: 31
  From24 : From  Commented=on  GotoTag=Lpower_TA  TagVisibility=global
  From25 : From  Commented=on  GotoTag=Rpower_TA  TagVisibility=global
  From26 : From  Commented=on  GotoTag=Lpower_HFL  TagVisibility=global
  From27 : From  Commented=on  GotoTag=Lpower_VAS  TagVisibility=global
  From28 : From  Commented=on  GotoTag=Rpower_HFL  TagVisibility=global
  From29 : From  Commented=on  GotoTag=Lpower_GAS  TagVisibility=global
  From30 : From  Commented=on  GotoTag=Rpower_VAS  TagVisibility=global
  From31 : From  Commented=on  GotoTag=Lpower_SOL  TagVisibility=global
  From32 : From  Commented=on  GotoTag=Lpower_HAM  TagVisibility=global
  From33 : From  Commented=on  GotoTag=Rpower_GAS  TagVisibility=global
  From34 : From  Commented=on  GotoTag=Lpower_GLU  TagVisibility=global
  From43 : From  Commented=on  GotoTag=LStimHFL  TagVisibility=global
  From44 : From  Commented=on  GotoTag=LStimGLU  TagVisibility=global
  From45 : From  Commented=on  GotoTag=LStimHAM  TagVisibility=global
  From46 : From  Commented=on  GotoTag=LStimVAS  TagVisibility=global
  From47 : From  Commented=on  GotoTag=LStimGAS  TagVisibility=global
  From51 : From  Commented=on  GotoTag=LStimTA  TagVisibility=global
  From52 : From  Commented=on  GotoTag=LStimSOL  TagVisibility=global
  From53 : From  Commented=on  GotoTag=RStimSOL  TagVisibility=global
  From54 : From  Commented=on  GotoTag=RStimTA  TagVisibility=global
  From55 : From  Commented=on  GotoTag=RStimGAS  TagVisibility=global
  From56 : From  Commented=on  GotoTag=RStimVAS  TagVisibility=global
  From57 : From  Commented=on  GotoTag=RStimHAM  TagVisibility=global
  From58 : From  Commented=on  GotoTag=RStimGLU  TagVisibility=global
  From59 : From  Commented=on  GotoTag=RStimHFL  TagVisibility=global
  From60 : From  Commented=on  GotoTag=LStimRF  TagVisibility=global
  From61 : From  Commented=on  GotoTag=LStance  TagVisibility=global
  From62 : From  Commented=on  GotoTag=RStance  TagVisibility=global
  From65 : From  Commented=on  GotoTag=Rpower_SOL  TagVisibility=global
  From66 : From  Commented=on  GotoTag=Rpower_HAM  TagVisibility=global
  From67 : From  Commented=on  GotoTag=Rpower_GLU  TagVisibility=global
  From68 : From  Commented=on  GotoTag=Rpower_HAMCut
  From75 : From  Commented=on  GotoTag=LStimBFSH  TagVisibility=global
  From76 : From  Commented=on  GotoTag=RStimRF  TagVisibility=global
  From77 : From  Commented=on  GotoTag=RStimBFSH  TagVisibility=global
  Mux : Mux  Inputs=11
  Mux1 : Mux
  Mux2 : Mux  Commented=on  Inputs=15
  Mux3 : Mux  Inputs=9
  Mux4 : Mux  Commented=on  Inputs=18
  Mux5 : Mux  Commented=on  Inputs=2
  Mux6 : Mux  Inputs=2
  Mux7 : Mux  Inputs=2
  Mux8 : Mux  Inputs=8
  Mux9 : Mux  Inputs=18
  Selector{1..4,6..9} (8 alike) : Selector  InputPortWidth=3  IndexOptions=Index vector (dialog)  Indices=[1 3]  OutputSizes=1
  Selector10 : Selector  InputPortWidth=6  IndexOptions=Index vector (dialog)  Indices=[1 3]  OutputSizes=1
  Selector11 : Selector  InputPortWidth=6  IndexOptions=Index vector (dialog)  Indices=[1 3]  OutputSizes=1
  Selector5 : Selector  InputPortWidth=6  IndexOptions=Index vector (dialog)  Indices=[1 3]  OutputSizes=1
  To Workspace : ToWorkspace  VariableName=animData2D  SaveFormat=Structure With Time  SampleTime=1/30
  To Workspace1 : ToWorkspace  VariableName=HATPosVel  SaveFormat=Structure With Time  SampleTime=dt_visual
  To Workspace10 : ToWorkspace  VariableName=TargetAngles  SaveFormat=Structure With Time  SampleTime=dt_visual
  To Workspace2 : ToWorkspace  Commented=on  VariableName=musculoPowerData  SaveFormat=Structure With Time  SampleTime=dt_visual
  To Workspace3 : ToWorkspace  VariableName=angularData  SaveFormat=Structure With Time  SampleTime=dt_visual
  To Workspace4 : ToWorkspace  Commented=on  VariableName=musculoStimData  SaveFormat=Structure With Time  SampleTime=dt_visual
  To Workspace5 : ToWorkspace  VariableName=GRFData  SaveFormat=Structure With Time  SampleTime=dt_visual
  To Workspace6 : ToWorkspace  Commented=on  VariableName=StanceData  SaveFormat=Structure With Time  SampleTime=1/30
  To Workspace7 : ToWorkspace  VariableName=GaitPhaseData  SaveFormat=Structure With Time  SampleTime=dt_visual
  To Workspace8 : ToWorkspace  VariableName=jointTorquesData  SaveFormat=Structure With Time  SampleTime=dt_visual
  To Workspace9 : ToWorkspace  VariableName=musculoData  SaveFormat=Structure With Time  SampleTime=dt_visual
  wires:
  [RAnklePos] -> Selector3/1
  [RKneePos] -> Selector4/1
  [RHipPosVel] -> Selector5/1
  [HATPosVel] -> Selector11/1
  [LHeelPos] -> Selector7/1
  [LBallPos] -> Selector6/1
  [LAnklePos] -> Selector8/1
  [LKneePos] -> Selector9/1
  [LHipPosVel] -> Selector10/1
  Selector11/1 -> Mux/1
  Selector3/1 -> Mux/9
  Selector4/1 -> Mux/8
  Selector5/1 -> Mux/7
  Selector7/1 -> Mux/6
  Selector6/1 -> Mux/5
  Selector8/1 -> Mux/4
  Selector9/1 -> Mux/3
  Selector10/1 -> Mux/2
  Mux/1 -> To Workspace/1
  [RHeelPos] -> Selector2/1
  [RBallPos] -> Selector1/1
  Selector2/1 -> Mux/11
  Selector1/1 -> Mux/10
  From61/1 -> Mux5/1
  From75/1 -> Mux4/6
  Mux4/1 -> To Workspace4/1
  [RphiANDdphiAnkle] -> Mux3/7
  Mux5/1 -> To Workspace6/1
  Mux6/1 -> To Workspace5/1
  From76/1 -> Mux4/13
  [RGRF] -> Mux6/2
  [phiANDdphiHAT] -> Mux3/1
  From51/1 -> Mux4/9
  Mux3/1 -> To Workspace3/1
  [LphiANDdphiAnkle] -> Mux3/6
  From58/1 -> Mux4/11
  [LphiANDdphiKnee] -> Mux3/4
  From57/1 -> Mux4/12
  From77/1 -> Mux4/15
  [LGRF] -> Mux6/1
  From56/1 -> Mux4/14
  [LphiANDdphiHip] -> Mux3/2
  From52/1 -> Mux4/8
  [RphiANDdphiKnee] -> Mux3/5
  From45/1 -> Mux4/3
  From43/1 -> Mux4/1
  From46/1 -> Mux4/5
  From59/1 -> Mux4/10
  From47/1 -> Mux4/7
  From44/1 -> Mux4/2
  From62/1 -> Mux5/2
  [RphiANDdphiHip] -> Mux3/3
  From60/1 -> Mux4/4
  [rightLegState] -> Mux7/2
  Mux7/1 -> To Workspace7/1
  [leftLegState] -> Mux7/1
  From31/1 -> Mux2/1
  From24/1 -> Mux2/2
  From29/1 -> Mux2/3
  From27/1 -> Mux2/4
  From32/1 -> Mux2/5
  From34/1 -> Mux2/6
  From26/1 -> Mux2/7
  From65/1 -> Mux2/8
  From25/1 -> Mux2/9
  From33/1 -> Mux2/10
  From30/1 -> Mux2/11
  From66/1 -> Mux2/12
  From67/1 -> Mux2/13
  From28/1 -> Mux2/14
  From68/1 -> Mux2/15
  Mux2/1 -> To Workspace2/1
  Mux8/1 -> To Workspace8/1
  [LHipMoment] -> Mux8/1
  [LKneeMoment] -> Mux8/2
  [LAnkleMoment] -> Mux8/3
  [RHipMoment] -> Mux8/4
  [RKneeMoment] -> Mux8/5
  [RAnkleMoment] -> Mux8/6
  From55/1 -> Mux4/16
  From53/1 -> Mux4/17
  From54/1 -> Mux4/18
  Mux9/1 -> To Workspace9/1
  [RdynHAM] -> Mux9/12
  [LdynHFL] -> Mux9/1
  [RdynGLU] -> Mux9/11
  [RdynVAS] -> Mux9/14
  [LdynBFSH] -> Mux9/6
  [RdynGAS] -> Mux9/16
  [RdynBFSH] -> Mux9/15
  [LdynVAS] -> Mux9/5
  [LdynGAS] -> Mux9/7
  [LdynSOL] -> Mux9/8
  [LdynRF] -> Mux9/4
  [LdynHAM] -> Mux9/3
  [LdynGLU] -> Mux9/2
  [LdynTA] -> Mux9/9
  [RdynRF] -> Mux9/13
  [RdynHFL] -> Mux9/10
  [RdynSOL] -> Mux9/17
  [RdynTA] -> Mux9/18
  [LHipMomentR] -> Mux8/7
  [RHipMomentR] -> Mux8/8
  [LthetaANDdthetaHipR] -> Mux3/8
  [RthetaANDdthetaHipR] -> Mux3/9
  [HATPosVel] -> To Workspace1/1
  [Lalpha_tgt] -> Mux1/1
  [LhipR_tgt] -> Mux1/2
  [Ralpha_tgt] -> Mux1/3
  [RhipR_tgt] -> Mux1/4
  Mux1/1 -> To Workspace10/1

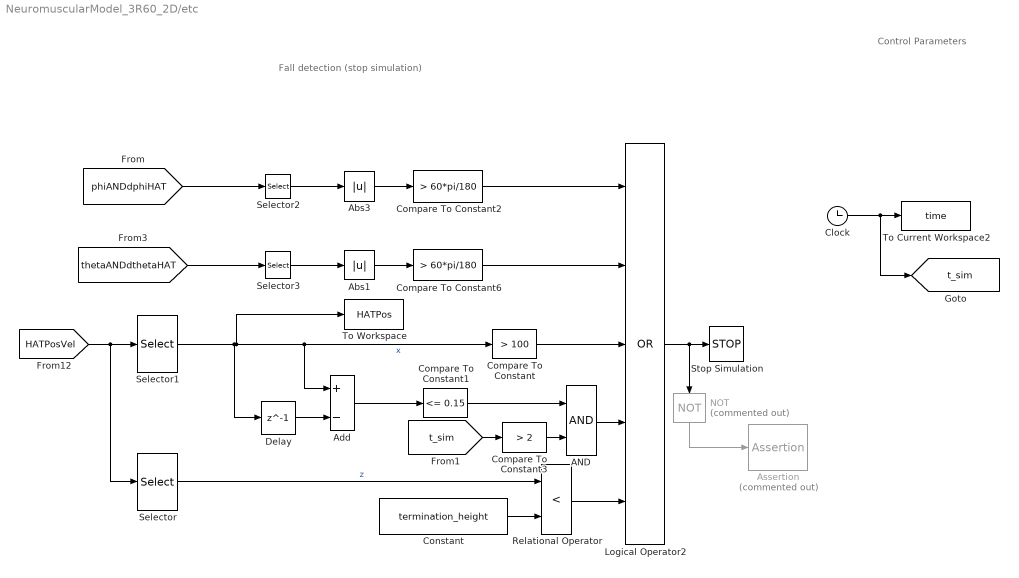
== system NeuromuscularModel_3R60_2D/etc ==
  note: Fall detection
      | (stop simulation)
  note: Control Parameters
  AND : Logic  AllPortsSameDT=off  OutDataTypeStr=boolean
  Abs1 : Abs
  Abs3 : Abs
  Add : Sum  Inputs=+-
  Assertion : Assertion  Commented=on  StopWhenAssertionFail=off
  Clock : Clock
  Compare To Constant : simulink/Logic and Bit Operations/Compare To Constant  relop=>  const=100  OutDataTypeStr=boolean
  Compare To Constant1 : simulink/Logic and Bit Operations/Compare To Constant  relop=<=  const=0.15  OutDataTypeStr=boolean
  Compare To Constant2 : simulink/Logic and Bit Operations/Compare To Constant  relop=>  const=60*pi/180  OutDataTypeStr=boolean
  Compare To Constant3 : simulink/Logic and Bit Operations/Compare To Constant  relop=>  const=2  OutDataTypeStr=boolean
  Compare To Constant6 : simulink/Logic and Bit Operations/Compare To Constant  relop=>  const=60*pi/180  OutDataTypeStr=boolean
  Constant : Constant  Value=termination_height
  Delay : Delay  DelayLength=1  SampleTime=1
  Logical Operator2 : Logic  Operator=OR  Inputs=5  AllPortsSameDT=off  OutDataTypeStr=boolean
  NOT : Logic  Commented=on  Operator=NOT  AllPortsSameDT=off  OutDataTypeStr=boolean
  Relational Operator : RelationalOperator  Operator=<  OutDataTypeStr=boolean  RndMeth=Nearest
  Selector : Selector  InputPortWidth=6  IndexOptions=Index vector (dialog)  Indices=[3]  OutputSizes=1
  Selector1 : Selector  InputPortWidth=6  IndexOptions=Index vector (dialog)  Indices=[1]  OutputSizes=1
  Selector2 : Selector  InputPortWidth=2  IndexOptions=Index vector (dialog)  Indices=[1]  OutputSizes=1
  Selector3 : Selector  InputPortWidth=2  IndexOptions=Index vector (dialog)  Indices=[1]  OutputSizes=1
  Stop Simulation : Stop
  To Current Workspace2 : ToWorkspace  VariableName=time  SampleTime=-1
      settings: MaxDataPoints=1
  To Workspace : ToWorkspace  VariableName=HATPos  SampleTime=-1
      settings: MaxDataPoints=1
  tag scope: t_sim=global
  wires:
  Selector2/1 -> Abs3/1
  Abs3/1 -> Compare To Constant2/1
  Compare To Constant2/1 -> Logical Operator2/1
  Logical Operator2/1 -> Stop Simulation/1, NOT/1
  Selector3/1 -> Abs1/1
  Abs1/1 -> Compare To Constant6/1
  Compare To Constant6/1 -> Logical Operator2/2
  Compare To Constant/1 -> Logical Operator2/3
  Selector/1 -> Relational Operator/1  "z"
  Selector1/1 -> To Workspace/1, Add/1, Compare To Constant/1, Delay/1  "x"
  Constant/1 -> Relational Operator/2
  Relational Operator/1 -> Logical Operator2/5
  [HATPosVel] -> Selector/1, Selector1/1
  Clock/1 -> [t_sim], To Current Workspace2/1
  [phiANDdphiHAT] -> Selector2/1
  [thetaANDdthetaHAT] -> Selector3/1
  Add/1 -> Compare To Constant1/1
  Compare To Constant1/1 -> AND/1
  Delay/1 -> Add/2
  AND/1 -> Logical Operator2/4
  [t_sim] -> Compare To Constant3/1
  Compare To Constant3/1 -> AND/2
  NOT/1 -> Assertion/1

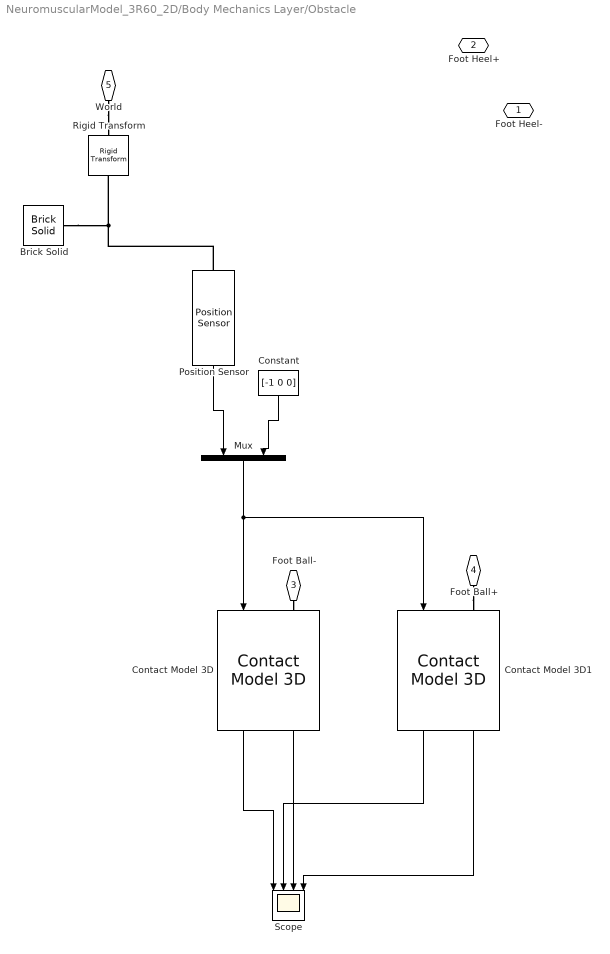
== system NeuromuscularModel_3R60_2D/Body Mechanics Layer/Obstacle ==
  Brick Solid : sm_lib/Body Elements/Brick Solid  GraphicAmbientColor=[0.15 0.15 0.15 1.0]  BasedOnType=Mass  BrickDimensions=[obstacle_depth obstacle_height obstacle_width]  BrickDimensionUnits=m  CenterOfMass=[0 0 0]  CenterOfMassUnits=m  GraphicDiffuseColor=[0.6 1.0 0.2]  Density=1000  DensityUnits=kg/m^3  DoExposeReferenceFrame=on  GraphicEmissiveColor=[0.0 0.0 0.0 1.0]  ExportEntireGeometry=off  SerializedFrames=<Frames/>  MarkerShape=Sphere  MarkerSize=10  GraphicType=FromGeometry  InertiaType=CalculateFromGeometry  Mass=0  MassUnits=kg  MomentsOfInertia=[1 1 1]  MomentsOfInertiaUnits=kg*m^2  GraphicOpacity=1.0  ProductsOfInertia=[0 0 0]  ProductsOfInertiaUnits=kg*m^2  GraphicShininess=75  GraphicSpecularColor=[0.5 0.5 0.5 1.0]  GraphicVisPropType=SimpleVisualProperties
  Constant : Constant  Value=[-1 0 0]
  Contact Model 3D : NeuroMuscularLibrary/Contact Model 3D  SystemSampleTime=-1  Latency=0  AutoFrameSizeCalculation=off
  Contact Model 3D1 : NeuroMuscularLibrary/Contact Model 3D  SystemSampleTime=-1  Latency=0  AutoFrameSizeCalculation=off
  Mux : Mux  Inputs=[3 3]
  Position Sensor : NeuroMuscularLibrary/Position Sensor  SystemSampleTime=-1  Latency=0  AutoFrameSizeCalculation=off
  Rigid Transform : sm_lib/Frames and Transforms/Rigid Transform  TranslationMethod=Cartesian  TranslationStandardOffset=0  TranslationLengthUnit=m  TranslationStandardAxis=+Z  TranslationCartesianOffset=[(obstacle_x+obstacle_depth/2) obstacle_height/2 0]  TranslationROffset=0  TranslationROffsetUnits=m  TranslationZOffset=0  TranslationZOffsetUnits=m  TranslationThetaOffset=0  TranslationThetaOffsetUnits=deg  RotationMethod=None  RotationAngleUnits=deg  RotationStandardAxis=+Z  RotationAngle=0.0  RotationArbitraryAxis=[0 0 1]  FollAlignAxisA=+X  BaseAlignAxisA=+Y  FollAlignAxisB=+Y  BaseAlignAxisB=+Z  RotationSequenceAxes=FollowerAxes  RotationSequence=XYX  RotationSequenceAngles=[0 0 0]  RotationSequenceAnglesUnits=deg  RotationMatrix=[1 0 0; 0 1 0; 0 0 1]
  Scope : Scope  NumInputPorts=4
  Foot Heel- : PMIOPort  Side=Left
  Foot Heel+ : PMIOPort  Port=2  Side=Left
  Foot Ball- : PMIOPort  Port=3  Side=Left
  Foot Ball+ : PMIOPort  Port=4  Side=Left
  World : PMIOPort  Port=5  Side=Left
  wires:
  Mux/1 -> Contact Model 3D1/1, Contact Model 3D/1
  Position Sensor/1 -> Mux/1
  Constant/1 -> Mux/2
  Contact Model 3D/2 -> Scope/3
  Contact Model 3D1/2 -> Scope/4
  Contact Model 3D1/1 -> Scope/2
  Contact Model 3D/1 -> Scope/1
  connections:
  Brick Solid/RConn1 -- Rigid Transform/RConn1 -- Position Sensor/LConn1
  Foot Ball-/RConn1 -- Contact Model 3D/LConn1
  World/RConn1 -- Rigid Transform/LConn1
  Foot Ball+/RConn1 -- Contact Model 3D1/LConn1
